simulink model "VCU_CS75_10_9_SteeringTorque"  (R2014a)
settings: Solver=FixedStepDiscrete  StartTime=0.0  StopTime=25  FixedStep=0.0005  RelTol=1e-3
undefined symbols (not defined in the file or in its folder): AutoDrivingReady, ecucoder_acal, I_SW01_L, LaterlAngleCommand, LDW, RemoteAcclPosition
libraries: simulink x880, ec5744lib x37
(part 22 of 30)

== system VCU_CS75_10_9_SteeringTorque/长安CS75底盘程序，20ms一次/Output/Subsystem/TransmitMessages4/ACC_3E5/ACC_takeoverRequesr ==
  ACC_takeoverRequesr : Inport
  ACC_takeoverRequesrRon : Rounding  Operator=round
  ACC_takeoverRequesr_1sat : Saturate  UpperLimit=8  LowerLimit=0
  ACC_takeoverRequesr_Convert : DataTypeConversion  OutDataTypeStr=uint8
  ACC_takeoverRequesr_Convert1 : DataTypeConversion  OutDataTypeStr=uint32
  ACC_takeoverRequesr_D : Product  Inputs=*/
  ACC_takeoverRequesr_F : Constant  OutDataTypeStr=single
  ACC_takeoverRequesr_L : simulink/Logic and Bit Operations/Bitwise Operator  logicop=AND  UseBitMask=on  BitMask=8  BitMaskRealWorld=Stored Integer
  ACC_takeoverRequesr_O : Constant  Value=0  OutDataTypeStr=single
  ACC_takeoverRequesr_S : ArithShift  BitShiftNumber=-3
  ACC_takeoverRequesr_sat : Saturate  UpperLimit=1  LowerLimit=0
  ACC_takeoverRequesr_st : Sum  Inputs=+-
  Constant{1..3,5..8} (7 alike) : Constant  Value=0  OutDataTypeStr=uint8
  output1 : Outport
  output2 : Outport  Port=2
  output3 : Outport  Port=3
  output4 : Outport  Port=4
  output5 : Outport  Port=5
  output6 : Outport  Port=6
  output7 : Outport  Port=7
  output8 : Outport  Port=8
  wires:
  Constant8/1 -> output8/1
  Constant7/1 -> output7/1
  Constant6/1 -> output6/1
  Constant5/1 -> output5/1
  Constant3/1 -> output3/1
  Constant2/1 -> output2/1
  Constant1/1 -> output1/1
  ACC_takeoverRequesr_Convert/1 -> output4/1
  ACC_takeoverRequesr_L/1 -> ACC_takeoverRequesr_Convert/1
  ACC_takeoverRequesr_Convert1/1 -> ACC_takeoverRequesr_L/1
  ACC_takeoverRequesr_1sat/1 -> ACC_takeoverRequesr_Convert1/1
  ACC_takeoverRequesr_S/1 -> ACC_takeoverRequesr_1sat/1
  ACC_takeoverRequesrRon/1 -> ACC_takeoverRequesr_S/1
  ACC_takeoverRequesr_D/1 -> ACC_takeoverRequesrRon/1
  ACC_takeoverRequesr_F/1 -> ACC_takeoverRequesr_D/2
  ACC_takeoverRequesr_st/1 -> ACC_takeoverRequesr_D/1
  ACC_takeoverRequesr_O/1 -> ACC_takeoverRequesr_st/2
  ACC_takeoverRequesr_sat/1 -> ACC_takeoverRequesr_st/1
  ACC_takeoverRequesr/1 -> ACC_takeoverRequesr_sat/1

== system VCU_CS75_10_9_SteeringTorque/长安CS75底盘程序，20ms一次/Output/Subsystem/TransmitMessages4/ACC_3E5/CRC ==
  CRC : Inport
  CRCRon : Rounding  Operator=round
  CRC_1sat : Saturate  UpperLimit=255  LowerLimit=0
  CRC_Convert : DataTypeConversion  OutDataTypeStr=uint8
  CRC_Convert1 : DataTypeConversion  OutDataTypeStr=uint32
  CRC_D : Product  Inputs=*/
  CRC_F : Constant  OutDataTypeStr=single
  CRC_L : simulink/Logic and Bit Operations/Bitwise Operator  logicop=AND  UseBitMask=on  BitMask=255  BitMaskRealWorld=Stored Integer
  CRC_O : Constant  Value=0  OutDataTypeStr=single
  CRC_S : ArithShift
  CRC_sat : Saturate  UpperLimit=0  LowerLimit=0
  CRC_st : Sum  Inputs=+-
  Constant{1..7} (7 alike) : Constant  Value=0  OutDataTypeStr=uint8
  output1 : Outport
  output2 : Outport  Port=2
  output3 : Outport  Port=3
  output4 : Outport  Port=4
  output5 : Outport  Port=5
  output6 : Outport  Port=6
  output7 : Outport  Port=7
  output8 : Outport  Port=8
  wires:
  Constant7/1 -> output7/1
  Constant6/1 -> output6/1
  Constant5/1 -> output5/1
  Constant4/1 -> output4/1
  Constant3/1 -> output3/1
  Constant2/1 -> output2/1
  Constant1/1 -> output1/1
  CRC_Convert/1 -> output8/1
  CRC_L/1 -> CRC_Convert/1
  CRC_Convert1/1 -> CRC_L/1
  CRC_1sat/1 -> CRC_Convert1/1
  CRC_S/1 -> CRC_1sat/1
  CRCRon/1 -> CRC_S/1
  CRC_D/1 -> CRCRon/1
  CRC_F/1 -> CRC_D/2
  CRC_st/1 -> CRC_D/1
  CRC_O/1 -> CRC_st/2
  CRC_sat/1 -> CRC_st/1
  CRC/1 -> CRC_sat/1

== system VCU_CS75_10_9_SteeringTorque/长安CS75底盘程序，20ms一次/Output/Subsystem/TransmitMessages4/ACC_3E5/RollingConter ==
  RollingConter : Inport
  Constant{1..6,8} (7 alike) : Constant  Value=0  OutDataTypeStr=uint8
  RollingConterRon : Rounding  Operator=round
  RollingConter_1sat : Saturate  UpperLimit=15  LowerLimit=0
  RollingConter_Convert : DataTypeConversion  OutDataTypeStr=uint8
  RollingConter_Convert1 : DataTypeConversion  OutDataTypeStr=uint32
  RollingConter_D : Product  Inputs=*/
  RollingConter_F : Constant  OutDataTypeStr=single
  RollingConter_L : simulink/Logic and Bit Operations/Bitwise Operator  logicop=AND  UseBitMask=on  BitMask=15  BitMaskRealWorld=Stored Integer
  RollingConter_O : Constant  Value=0  OutDataTypeStr=single
  RollingConter_S : ArithShift
  RollingConter_sat : Saturate  UpperLimit=0  LowerLimit=0
  RollingConter_st : Sum  Inputs=+-
  output1 : Outport
  output2 : Outport  Port=2
  output3 : Outport  Port=3
  output4 : Outport  Port=4
  output5 : Outport  Port=5
  output6 : Outport  Port=6
  output7 : Outport  Port=7
  output8 : Outport  Port=8
  wires:
  Constant8/1 -> output8/1
  Constant6/1 -> output6/1
  Constant5/1 -> output5/1
  Constant4/1 -> output4/1
  Constant3/1 -> output3/1
  Constant2/1 -> output2/1
  Constant1/1 -> output1/1
  RollingConter_Convert/1 -> output7/1
  RollingConter_L/1 -> RollingConter_Convert/1
  RollingConter_Convert1/1 -> RollingConter_L/1
  RollingConter_1sat/1 -> RollingConter_Convert1/1
  RollingConter_S/1 -> RollingConter_1sat/1
  RollingConterRon/1 -> RollingConter_S/1
  RollingConter_D/1 -> RollingConterRon/1
  RollingConter_F/1 -> RollingConter_D/2
  RollingConter_st/1 -> RollingConter_D/1
  RollingConter_O/1 -> RollingConter_st/2
  RollingConter_sat/1 -> RollingConter_st/1
  RollingConter/1 -> RollingConter_sat/1

== system VCU_CS75_10_9_SteeringTorque/长安CS75底盘程序，20ms一次/Output/Subsystem/TransmitMessages5/ACC_3F5/ACC_AEBTargetLatRange ==
  ACC_AEBTargetLatRange : Inport
  ACC_AEBTargetLatRangeBitCov : DataTypeConversion  OutDataTypeStr=uint8
  ACC_AEBTargetLatRangeCOV : DataTypeConversion  OutDataTypeStr=uint8
  ACC_AEBTargetLatRangeRon : Rounding  Operator=round
  ACC_AEBTargetLatRange_1sat : Saturate  UpperLimit=16368  LowerLimit=0
  ACC_AEBTargetLatRange_And : simulink/Logic and Bit Operations/Bitwise Operator  logicop=AND  UseBitMask=off  NumInputPorts=2  BitMask=bin2dec('11011001')  BitMaskRealWorld=Stored Integer
  ACC_AEBTargetLatRange_And_C : Constant  Value=255  OutDataTypeStr=uint32
  ACC_AEBTargetLatRange_Convert : DataTypeConversion  OutDataTypeStr=uint32
  ACC_AEBTargetLatRange_D : Product  Inputs=*/
  ACC_AEBTargetLatRange_D1 : Product  Inputs=*/
  ACC_AEBTargetLatRange_F : Constant  Value=0.1  OutDataTypeStr=single
  ACC_AEBTargetLatRange_L : simulink/Logic and Bit Operations/Bitwise Operator  logicop=AND  UseBitMask=on  BitMask=16368  BitMaskRealWorld=Stored Integer
  ACC_AEBTargetLatRange_O : Constant  Value=-50  OutDataTypeStr=single
  ACC_AEBTargetLatRange_S : ArithShift  BitShiftNumber=-4
  ACC_AEBTargetLatRange_sat : Saturate  UpperLimit=52.3  LowerLimit=-50
  ACC_AEBTargetLatRange_st : Sum  Inputs=+-
  ACC_AEBTargetLatRangeoutput3_C : Constant  Value=256
  Constant{1..2,5..8} (6 alike) : Constant  Value=0  OutDataTypeStr=uint8
  output1 : Outport
  output2 : Outport  Port=2
  output3 : Outport  Port=3
  output4 : Outport  Port=4
  output5 : Outport  Port=5
  output6 : Outport  Port=6
  output7 : Outport  Port=7
  output8 : Outport  Port=8
  wires:
  ACC_AEBTargetLatRange/1 -> ACC_AEBTargetLatRange_sat/1
  ACC_AEBTargetLatRange_sat/1 -> ACC_AEBTargetLatRange_st/1
  ACC_AEBTargetLatRange_O/1 -> ACC_AEBTargetLatRange_st/2
  ACC_AEBTargetLatRange_st/1 -> ACC_AEBTargetLatRange_D/1
  ACC_AEBTargetLatRange_F/1 -> ACC_AEBTargetLatRange_D/2
  ACC_AEBTargetLatRange_D/1 -> ACC_AEBTargetLatRangeRon/1
  ACC_AEBTargetLatRangeRon/1 -> ACC_AEBTargetLatRange_S/1
  ACC_AEBTargetLatRange_S/1 -> ACC_AEBTargetLatRange_1sat/1
  ACC_AEBTargetLatRange_1sat/1 -> ACC_AEBTargetLatRange_Convert/1
  ACC_AEBTargetLatRange_Convert/1 -> ACC_AEBTargetLatRange_L/1
  ACC_AEBTargetLatRange_L/1 -> ACC_AEBTargetLatRange_D1/1, ACC_AEBTargetLatRange_And/1
  ACC_AEBTargetLatRangeoutput3_C/1 -> ACC_AEBTargetLatRange_D1/2
  ACC_AEBTargetLatRange_D1/1 -> ACC_AEBTargetLatRangeCOV/1
  ACC_AEBTargetLatRangeCOV/1 -> output3/1
  ACC_AEBTargetLatRange_And_C/1 -> ACC_AEBTargetLatRange_And/2
  ACC_AEBTargetLatRange_And/1 -> ACC_AEBTargetLatRangeBitCov/1
  ACC_AEBTargetLatRangeBitCov/1 -> output4/1
  Constant1/1 -> output1/1
  Constant2/1 -> output2/1
  Constant5/1 -> output5/1
  Constant6/1 -> output6/1
  Constant7/1 -> output7/1
  Constant8/1 -> output8/1

== system VCU_CS75_10_9_SteeringTorque/长安CS75底盘程序，20ms一次/Output/Subsystem/TransmitMessages5/ACC_3F5/ACC_AEBTargetLngRange ==
  ACC_AEBTargetLngRange : Inport
  ACC_AEBTargetLngRangeBitCov : DataTypeConversion  OutDataTypeStr=uint8
  ACC_AEBTargetLngRangeCOV : DataTypeConversion  OutDataTypeStr=uint8
  ACC_AEBTargetLngRangeRon : Rounding  Operator=round
  ACC_AEBTargetLngRange_1sat : Saturate  UpperLimit=65408  LowerLimit=0
  ACC_AEBTargetLngRange_And : simulink/Logic and Bit Operations/Bitwise Operator  logicop=AND  UseBitMask=off  NumInputPorts=2  BitMask=bin2dec('11011001')  BitMaskRealWorld=Stored Integer
  ACC_AEBTargetLngRange_And_C : Constant  Value=255  OutDataTypeStr=uint32
  ACC_AEBTargetLngRange_Convert : DataTypeConversion  OutDataTypeStr=uint32
  ACC_AEBTargetLngRange_D : Product  Inputs=*/
  ACC_AEBTargetLngRange_D1 : Product  Inputs=*/
  ACC_AEBTargetLngRange_F : Constant  Value=0.5  OutDataTypeStr=single
  ACC_AEBTargetLngRange_L : simulink/Logic and Bit Operations/Bitwise Operator  logicop=AND  UseBitMask=on  BitMask=65408  BitMaskRealWorld=Stored Integer
  ACC_AEBTargetLngRange_O : Constant  Value=0  OutDataTypeStr=single
  ACC_AEBTargetLngRange_S : ArithShift  BitShiftNumber=-7
  ACC_AEBTargetLngRange_sat : Saturate  UpperLimit=0  LowerLimit=0
  ACC_AEBTargetLngRange_st : Sum  Inputs=+-
  ACC_AEBTargetLngRangeoutput1_C : Constant  Value=256
  Constant{3..8} (6 alike) : Constant  Value=0  OutDataTypeStr=uint8
  output1 : Outport
  output2 : Outport  Port=2
  output3 : Outport  Port=3
  output4 : Outport  Port=4
  output5 : Outport  Port=5
  output6 : Outport  Port=6
  output7 : Outport  Port=7
  output8 : Outport  Port=8
  wires:
  ACC_AEBTargetLngRange/1 -> ACC_AEBTargetLngRange_sat/1
  ACC_AEBTargetLngRange_sat/1 -> ACC_AEBTargetLngRange_st/1
  ACC_AEBTargetLngRange_O/1 -> ACC_AEBTargetLngRange_st/2
  ACC_AEBTargetLngRange_st/1 -> ACC_AEBTargetLngRange_D/1
  ACC_AEBTargetLngRange_F/1 -> ACC_AEBTargetLngRange_D/2
  ACC_AEBTargetLngRange_D/1 -> ACC_AEBTargetLngRangeRon/1
  ACC_AEBTargetLngRangeRon/1 -> ACC_AEBTargetLngRange_S/1
  ACC_AEBTargetLngRange_S/1 -> ACC_AEBTargetLngRange_1sat/1
  ACC_AEBTargetLngRange_1sat/1 -> ACC_AEBTargetLngRange_Convert/1
  ACC_AEBTargetLngRange_Convert/1 -> ACC_AEBTargetLngRange_L/1
  ACC_AEBTargetLngRange_L/1 -> ACC_AEBTargetLngRange_D1/1, ACC_AEBTargetLngRange_And/1
  ACC_AEBTargetLngRangeoutput1_C/1 -> ACC_AEBTargetLngRange_D1/2
  ACC_AEBTargetLngRange_D1/1 -> ACC_AEBTargetLngRangeCOV/1
  ACC_AEBTargetLngRangeCOV/1 -> output1/1
  ACC_AEBTargetLngRange_And_C/1 -> ACC_AEBTargetLngRange_And/2
  ACC_AEBTargetLngRange_And/1 -> ACC_AEBTargetLngRangeBitCov/1
  ACC_AEBTargetLngRangeBitCov/1 -> output2/1
  Constant3/1 -> output3/1
  Constant4/1 -> output4/1
  Constant5/1 -> output5/1
  Constant6/1 -> output6/1
  Constant7/1 -> output7/1
  Constant8/1 -> output8/1

== system VCU_CS75_10_9_SteeringTorque/长安CS75底盘程序，20ms一次/Output/Subsystem/TransmitMessages5/ACC_3F5/ACC_AEBTargetRelSpeed ==
  ACC_AEBTargetRelSpeed : Inport
  ACC_AEBTargetRelSpeedBitCov : DataTypeConversion  OutDataTypeStr=uint8
  ACC_AEBTargetRelSpeedCOV : DataTypeConversion  OutDataTypeStr=uint8
  ACC_AEBTargetRelSpeedRon : Rounding  Operator=round
  ACC_AEBTargetRelSpeed_1sat : Saturate  UpperLimit=32704  LowerLimit=0
  ACC_AEBTargetRelSpeed_And : simulink/Logic and Bit Operations/Bitwise Operator  logicop=AND  UseBitMask=off  NumInputPorts=2  BitMask=bin2dec('11011001')  BitMaskRealWorld=Stored Integer
  ACC_AEBTargetRelSpeed_And_C : Constant  Value=255  OutDataTypeStr=uint32
  ACC_AEBTargetRelSpeed_Convert : DataTypeConversion  OutDataTypeStr=uint32
  ACC_AEBTargetRelSpeed_D : Product  Inputs=*/
  ACC_AEBTargetRelSpeed_D1 : Product  Inputs=*/
  ACC_AEBTargetRelSpeed_F : Constant  OutDataTypeStr=single
  ACC_AEBTargetRelSpeed_L : simulink/Logic and Bit Operations/Bitwise Operator  logicop=AND  UseBitMask=on  BitMask=32704  BitMaskRealWorld=Stored Integer
  ACC_AEBTargetRelSpeed_O : Constant  Value=0  OutDataTypeStr=single
  ACC_AEBTargetRelSpeed_S : ArithShift  BitShiftNumber=-6
  ACC_AEBTargetRelSpeed_sat : Saturate  UpperLimit=0  LowerLimit=0
  ACC_AEBTargetRelSpeed_st : Sum  Inputs=+-
  ACC_AEBTargetRelSpeedoutput2_C : Constant  Value=256
  Constant{1,4..8} (6 alike) : Constant  Value=0  OutDataTypeStr=uint8
  output1 : Outport
  output2 : Outport  Port=2
  output3 : Outport  Port=3
  output4 : Outport  Port=4
  output5 : Outport  Port=5
  output6 : Outport  Port=6
  output7 : Outport  Port=7
  output8 : Outport  Port=8
  wires:
  ACC_AEBTargetRelSpeed/1 -> ACC_AEBTargetRelSpeed_sat/1
  ACC_AEBTargetRelSpeed_sat/1 -> ACC_AEBTargetRelSpeed_st/1
  ACC_AEBTargetRelSpeed_O/1 -> ACC_AEBTargetRelSpeed_st/2
  ACC_AEBTargetRelSpeed_st/1 -> ACC_AEBTargetRelSpeed_D/1
  ACC_AEBTargetRelSpeed_F/1 -> ACC_AEBTargetRelSpeed_D/2
  ACC_AEBTargetRelSpeed_D/1 -> ACC_AEBTargetRelSpeedRon/1
  ACC_AEBTargetRelSpeedRon/1 -> ACC_AEBTargetRelSpeed_S/1
  ACC_AEBTargetRelSpeed_S/1 -> ACC_AEBTargetRelSpeed_1sat/1
  ACC_AEBTargetRelSpeed_1sat/1 -> ACC_AEBTargetRelSpeed_Convert/1
  ACC_AEBTargetRelSpeed_Convert/1 -> ACC_AEBTargetRelSpeed_L/1
  ACC_AEBTargetRelSpeed_L/1 -> ACC_AEBTargetRelSpeed_D1/1, ACC_AEBTargetRelSpeed_And/1
  ACC_AEBTargetRelSpeedoutput2_C/1 -> ACC_AEBTargetRelSpeed_D1/2
  ACC_AEBTargetRelSpeed_D1/1 -> ACC_AEBTargetRelSpeedCOV/1
  ACC_AEBTargetRelSpeedCOV/1 -> output2/1
  ACC_AEBTargetRelSpeed_And_C/1 -> ACC_AEBTargetRelSpeed_And/2
  ACC_AEBTargetRelSpeed_And/1 -> ACC_AEBTargetRelSpeedBitCov/1
  ACC_AEBTargetRelSpeedBitCov/1 -> output3/1
  Constant1/1 -> output1/1
  Constant4/1 -> output4/1
  Constant5/1 -> output5/1
  Constant6/1 -> output6/1
  Constant7/1 -> output7/1
  Constant8/1 -> output8/1

== system VCU_CS75_10_9_SteeringTorque/长安CS75底盘程序，20ms一次/Output/Subsystem/TransmitMessages5/ACC_3F5/ACC_HostPotentialTargetDetection ==
  ACC_HostPotentialTargetDetection : Inport
  ACC_HostPotentialTargetDetectionRon : Rounding  Operator=round
  ACC_HostPotentialTargetDetection_1sat : Saturate  UpperLimit=12  LowerLimit=0
  ACC_HostPotentialTargetDetection_Convert : DataTypeConversion  OutDataTypeStr=uint8
  ACC_HostPotentialTargetDetection_Convert1 : DataTypeConversion  OutDataTypeStr=uint32
  ACC_HostPotentialTargetDetection_D : Product  Inputs=*/
  ACC_HostPotentialTargetDetection_F : Constant  OutDataTypeStr=single
  ACC_HostPotentialTargetDetection_L : simulink/Logic and Bit Operations/Bitwise Operator  logicop=AND  UseBitMask=on  BitMask=12  BitMaskRealWorld=Stored Integer
  ACC_HostPotentialTargetDetection_O : Constant  Value=0  OutDataTypeStr=single
  ACC_HostPotentialTargetDetection_S : ArithShift  BitShiftNumber=-2
  ACC_HostPotentialTargetDetection_sat : Saturate  UpperLimit=3  LowerLimit=0
  ACC_HostPotentialTargetDetection_st : Sum  Inputs=+-
  Constant{1..3,5..8} (7 alike) : Constant  Value=0  OutDataTypeStr=uint8
  output1 : Outport
  output2 : Outport  Port=2
  output3 : Outport  Port=3
  output4 : Outport  Port=4
  output5 : Outport  Port=5
  output6 : Outport  Port=6
  output7 : Outport  Port=7
  output8 : Outport  Port=8
  wires:
  ACC_HostPotentialTargetDetection/1 -> ACC_HostPotentialTargetDetection_sat/1
  ACC_HostPotentialTargetDetection_sat/1 -> ACC_HostPotentialTargetDetection_st/1
  ACC_HostPotentialTargetDetection_O/1 -> ACC_HostPotentialTargetDetection_st/2
  ACC_HostPotentialTargetDetection_st/1 -> ACC_HostPotentialTargetDetection_D/1
  ACC_HostPotentialTargetDetection_F/1 -> ACC_HostPotentialTargetDetection_D/2
  ACC_HostPotentialTargetDetection_D/1 -> ACC_HostPotentialTargetDetectionRon/1
  ACC_HostPotentialTargetDetectionRon/1 -> ACC_HostPotentialTargetDetection_S/1
  ACC_HostPotentialTargetDetection_S/1 -> ACC_HostPotentialTargetDetection_1sat/1
  ACC_HostPotentialTargetDetection_1sat/1 -> ACC_HostPotentialTargetDetection_Convert1/1
  ACC_HostPotentialTargetDetection_Convert1/1 -> ACC_HostPotentialTargetDetection_L/1
  ACC_HostPotentialTargetDetection_L/1 -> ACC_HostPotentialTargetDetection_Convert/1
  ACC_HostPotentialTargetDetection_Convert/1 -> output4/1
  Constant1/1 -> output1/1
  Constant2/1 -> output2/1
  Constant3/1 -> output3/1
  Constant5/1 -> output5/1
  Constant6/1 -> output6/1
  Constant7/1 -> output7/1
  Constant8/1 -> output8/1

== system VCU_CS75_10_9_SteeringTorque/长安CS75底盘程序，20ms一次/Output/Subsystem/TransmitMessages5/ACC_3F5/ACC_HostPotentialTargetLatRng ==
  ACC_HostPotentialTargetLatRng : Inport
  ACC_HostPotentialTargetLatRngBitCov : DataTypeConversion  OutDataTypeStr=uint8
  ACC_HostPotentialTargetLatRngCOV : DataTypeConversion  OutDataTypeStr=uint8
  ACC_HostPotentialTargetLatRngRon : Rounding  Operator=round
  ACC_HostPotentialTargetLatRng_1sat : Saturate  UpperLimit=1023  LowerLimit=0
  ACC_HostPotentialTargetLatRng_And : simulink/Logic and Bit Operations/Bitwise Operator  logicop=AND  UseBitMask=off  NumInputPorts=2  BitMask=bin2dec('11011001')  BitMaskRealWorld=Stored Integer
  ACC_HostPotentialTargetLatRng_And_C : Constant  Value=255  OutDataTypeStr=uint32
  ACC_HostPotentialTargetLatRng_Convert : DataTypeConversion  OutDataTypeStr=uint32
  ACC_HostPotentialTargetLatRng_D : Product  Inputs=*/
  ACC_HostPotentialTargetLatRng_D1 : Product  Inputs=*/
  ACC_HostPotentialTargetLatRng_F : Constant  Value=0.1  OutDataTypeStr=single
  ACC_HostPotentialTargetLatRng_L : simulink/Logic and Bit Operations/Bitwise Operator  logicop=AND  UseBitMask=on  BitMask=1023  BitMaskRealWorld=Stored Integer
  ACC_HostPotentialTargetLatRng_O : Constant  Value=-50  OutDataTypeStr=single
  ACC_HostPotentialTargetLatRng_S : ArithShift
  ACC_HostPotentialTargetLatRng_sat : Saturate  UpperLimit=52.3  LowerLimit=-50
  ACC_HostPotentialTargetLatRng_st : Sum  Inputs=+-
  ACC_HostPotentialTargetLatRngoutput4_C : Constant  Value=256
  Constant{1..3,6..8} (6 alike) : Constant  Value=0  OutDataTypeStr=uint8
  output1 : Outport
  output2 : Outport  Port=2
  output3 : Outport  Port=3
  output4 : Outport  Port=4
  output5 : Outport  Port=5
  output6 : Outport  Port=6
  output7 : Outport  Port=7
  output8 : Outport  Port=8
  wires:
  ACC_HostPotentialTargetLatRng/1 -> ACC_HostPotentialTargetLatRng_sat/1
  ACC_HostPotentialTargetLatRng_sat/1 -> ACC_HostPotentialTargetLatRng_st/1
  ACC_HostPotentialTargetLatRng_O/1 -> ACC_HostPotentialTargetLatRng_st/2
  ACC_HostPotentialTargetLatRng_st/1 -> ACC_HostPotentialTargetLatRng_D/1
  ACC_HostPotentialTargetLatRng_F/1 -> ACC_HostPotentialTargetLatRng_D/2
  ACC_HostPotentialTargetLatRng_D/1 -> ACC_HostPotentialTargetLatRngRon/1
  ACC_HostPotentialTargetLatRngRon/1 -> ACC_HostPotentialTargetLatRng_S/1
  ACC_HostPotentialTargetLatRng_S/1 -> ACC_HostPotentialTargetLatRng_1sat/1
  ACC_HostPotentialTargetLatRng_1sat/1 -> ACC_HostPotentialTargetLatRng_Convert/1
  ACC_HostPotentialTargetLatRng_Convert/1 -> ACC_HostPotentialTargetLatRng_L/1
  ACC_HostPotentialTargetLatRng_L/1 -> ACC_HostPotentialTargetLatRng_D1/1, ACC_HostPotentialTargetLatRng_And/1
  ACC_HostPotentialTargetLatRngoutput4_C/1 -> ACC_HostPotentialTargetLatRng_D1/2
  ACC_HostPotentialTargetLatRng_D1/1 -> ACC_HostPotentialTargetLatRngCOV/1
  ACC_HostPotentialTargetLatRngCOV/1 -> output4/1
  ACC_HostPotentialTargetLatRng_And_C/1 -> ACC_HostPotentialTargetLatRng_And/2
  ACC_HostPotentialTargetLatRng_And/1 -> ACC_HostPotentialTargetLatRngBitCov/1
  ACC_HostPotentialTargetLatRngBitCov/1 -> output5/1
  Constant1/1 -> output1/1
  Constant2/1 -> output2/1
  Constant3/1 -> output3/1
  Constant6/1 -> output6/1
  Constant7/1 -> output7/1
  Constant8/1 -> output8/1

== system VCU_CS75_10_9_SteeringTorque/长安CS75底盘程序，20ms一次/Output/Subsystem/TransmitMessages5/ACC_3F5/ACC_HostPotentialTargetLngRng ==
  ACC_HostPotentialTargetLngRng : Inport
  ACC_HostPotentialTargetLngRngBitCov : DataTypeConversion  OutDataTypeStr=uint8
  ACC_HostPotentialTargetLngRngCOV : DataTypeConversion  OutDataTypeStr=uint8
  ACC_HostPotentialTargetLngRngRon : Rounding  Operator=round
  ACC_HostPotentialTargetLngRng_1sat : Saturate  UpperLimit=65408  LowerLimit=0
  ACC_HostPotentialTargetLngRng_And : simulink/Logic and Bit Operations/Bitwise Operator  logicop=AND  UseBitMask=off  NumInputPorts=2  BitMask=bin2dec('11011001')  BitMaskRealWorld=Stored Integer
  ACC_HostPotentialTargetLngRng_And_C : Constant  Value=255  OutDataTypeStr=uint32
  ACC_HostPotentialTargetLngRng_Convert : DataTypeConversion  OutDataTypeStr=uint32
  ACC_HostPotentialTargetLngRng_D : Product  Inputs=*/
  ACC_HostPotentialTargetLngRng_D1 : Product  Inputs=*/
  ACC_HostPotentialTargetLngRng_F : Constant  Value=0.5  OutDataTypeStr=single
  ACC_HostPotentialTargetLngRng_L : simulink/Logic and Bit Operations/Bitwise Operator  logicop=AND  UseBitMask=on  BitMask=65408  BitMaskRealWorld=Stored Integer
  ACC_HostPotentialTargetLngRng_O : Constant  Value=0  OutDataTypeStr=single
  ACC_HostPotentialTargetLngRng_S : ArithShift  BitShiftNumber=-7
  ACC_HostPotentialTargetLngRng_sat : Saturate  UpperLimit=255.5  LowerLimit=0
  ACC_HostPotentialTargetLngRng_st : Sum  Inputs=+-
  ACC_HostPotentialTargetLngRngoutput6_C : Constant  Value=256
  Constant{1..5,8} (6 alike) : Constant  Value=0  OutDataTypeStr=uint8
  output1 : Outport
  output2 : Outport  Port=2
  output3 : Outport  Port=3
  output4 : Outport  Port=4
  output5 : Outport  Port=5
  output6 : Outport  Port=6
  output7 : Outport  Port=7
  output8 : Outport  Port=8
  wires:
  ACC_HostPotentialTargetLngRng/1 -> ACC_HostPotentialTargetLngRng_sat/1
  ACC_HostPotentialTargetLngRng_sat/1 -> ACC_HostPotentialTargetLngRng_st/1
  ACC_HostPotentialTargetLngRng_O/1 -> ACC_HostPotentialTargetLngRng_st/2
  ACC_HostPotentialTargetLngRng_st/1 -> ACC_HostPotentialTargetLngRng_D/1
  ACC_HostPotentialTargetLngRng_F/1 -> ACC_HostPotentialTargetLngRng_D/2
  ACC_HostPotentialTargetLngRng_D/1 -> ACC_HostPotentialTargetLngRngRon/1
  ACC_HostPotentialTargetLngRngRon/1 -> ACC_HostPotentialTargetLngRng_S/1
  ACC_HostPotentialTargetLngRng_S/1 -> ACC_HostPotentialTargetLngRng_1sat/1
  ACC_HostPotentialTargetLngRng_1sat/1 -> ACC_HostPotentialTargetLngRng_Convert/1
  ACC_HostPotentialTargetLngRng_Convert/1 -> ACC_HostPotentialTargetLngRng_L/1
  ACC_HostPotentialTargetLngRng_L/1 -> ACC_HostPotentialTargetLngRng_D1/1, ACC_HostPotentialTargetLngRng_And/1
  ACC_HostPotentialTargetLngRngoutput6_C/1 -> ACC_HostPotentialTargetLngRng_D1/2
  ACC_HostPotentialTargetLngRng_D1/1 -> ACC_HostPotentialTargetLngRngCOV/1
  ACC_HostPotentialTargetLngRngCOV/1 -> output6/1
  ACC_HostPotentialTargetLngRng_And_C/1 -> ACC_HostPotentialTargetLngRng_And/2
  ACC_HostPotentialTargetLngRng_And/1 -> ACC_HostPotentialTargetLngRngBitCov/1
  ACC_HostPotentialTargetLngRngBitCov/1 -> output7/1
  Constant1/1 -> output1/1
  Constant2/1 -> output2/1
  Constant3/1 -> output3/1
  Constant4/1 -> output4/1
  Constant5/1 -> output5/1
  Constant8/1 -> output8/1

== system VCU_CS75_10_9_SteeringTorque/长安CS75底盘程序，20ms一次/Output/Subsystem/TransmitMessages5/ACC_3F5/ACC_HostPotentialTargetType ==
  ACC_HostPotentialTargetType : Inport
  ACC_HostPotentialTargetTypeRon : Rounding  Operator=round
  ACC_HostPotentialTargetType_1sat : Saturate  UpperLimit=112  LowerLimit=0
  ACC_HostPotentialTargetType_Convert : DataTypeConversion  OutDataTypeStr=uint8
  ACC_HostPotentialTargetType_Convert1 : DataTypeConversion  OutDataTypeStr=uint32
  ACC_HostPotentialTargetType_D : Product  Inputs=*/
  ACC_HostPotentialTargetType_F : Constant  OutDataTypeStr=single
  ACC_HostPotentialTargetType_L : simulink/Logic and Bit Operations/Bitwise Operator  logicop=AND  UseBitMask=on  BitMask=112  BitMaskRealWorld=Stored Integer
  ACC_HostPotentialTargetType_O : Constant  Value=0  OutDataTypeStr=single
  ACC_HostPotentialTargetType_S : ArithShift  BitShiftNumber=-4
  ACC_HostPotentialTargetType_sat : Saturate  UpperLimit=7  LowerLimit=0
  ACC_HostPotentialTargetType_st : Sum  Inputs=+-
  Constant{1..6,8} (7 alike) : Constant  Value=0  OutDataTypeStr=uint8
  output1 : Outport
  output2 : Outport  Port=2
  output3 : Outport  Port=3
  output4 : Outport  Port=4
  output5 : Outport  Port=5
  output6 : Outport  Port=6
  output7 : Outport  Port=7
  output8 : Outport  Port=8
  wires:
  ACC_HostPotentialTargetType/1 -> ACC_HostPotentialTargetType_sat/1
  ACC_HostPotentialTargetType_sat/1 -> ACC_HostPotentialTargetType_st/1
  ACC_HostPotentialTargetType_O/1 -> ACC_HostPotentialTargetType_st/2
  ACC_HostPotentialTargetType_st/1 -> ACC_HostPotentialTargetType_D/1
  ACC_HostPotentialTargetType_F/1 -> ACC_HostPotentialTargetType_D/2
  ACC_HostPotentialTargetType_D/1 -> ACC_HostPotentialTargetTypeRon/1
  ACC_HostPotentialTargetTypeRon/1 -> ACC_HostPotentialTargetType_S/1
  ACC_HostPotentialTargetType_S/1 -> ACC_HostPotentialTargetType_1sat/1
  ACC_HostPotentialTargetType_1sat/1 -> ACC_HostPotentialTargetType_Convert1/1
  ACC_HostPotentialTargetType_Convert1/1 -> ACC_HostPotentialTargetType_L/1
  ACC_HostPotentialTargetType_L/1 -> ACC_HostPotentialTargetType_Convert/1
  ACC_HostPotentialTargetType_Convert/1 -> output7/1
  Constant1/1 -> output1/1
  Constant2/1 -> output2/1
  Constant3/1 -> output3/1
  Constant4/1 -> output4/1
  Constant5/1 -> output5/1
  Constant6/1 -> output6/1
  Constant8/1 -> output8/1

== system VCU_CS75_10_9_SteeringTorque/长安CS75底盘程序，20ms一次/Output/Subsystem/TransmitMessages5/ACC_3F5/CRC ==
  CRC : Inport
  CRCRon : Rounding  Operator=round
  CRC_1sat : Saturate  UpperLimit=255  LowerLimit=0
  CRC_Convert : DataTypeConversion  OutDataTypeStr=uint8
  CRC_Convert1 : DataTypeConversion  OutDataTypeStr=uint32
  CRC_D : Product  Inputs=*/
  CRC_F : Constant  OutDataTypeStr=single
  CRC_L : simulink/Logic and Bit Operations/Bitwise Operator  logicop=AND  UseBitMask=on  BitMask=255  BitMaskRealWorld=Stored Integer
  CRC_O : Constant  Value=0  OutDataTypeStr=single
  CRC_S : ArithShift
  CRC_sat : Saturate  UpperLimit=0  LowerLimit=0
  CRC_st : Sum  Inputs=+-
  Constant{1..7} (7 alike) : Constant  Value=0  OutDataTypeStr=uint8
  output1 : Outport
  output2 : Outport  Port=2
  output3 : Outport  Port=3
  output4 : Outport  Port=4
  output5 : Outport  Port=5
  output6 : Outport  Port=6
  output7 : Outport  Port=7
  output8 : Outport  Port=8
  wires:
  CRC/1 -> CRC_sat/1
  CRC_sat/1 -> CRC_st/1
  CRC_O/1 -> CRC_st/2
  CRC_st/1 -> CRC_D/1
  CRC_F/1 -> CRC_D/2
  CRC_D/1 -> CRCRon/1
  CRCRon/1 -> CRC_S/1
  CRC_S/1 -> CRC_1sat/1
  CRC_1sat/1 -> CRC_Convert1/1
  CRC_Convert1/1 -> CRC_L/1
  CRC_L/1 -> CRC_Convert/1
  CRC_Convert/1 -> output8/1
  Constant1/1 -> output1/1
  Constant2/1 -> output2/1
  Constant3/1 -> output3/1
  Constant4/1 -> output4/1
  Constant5/1 -> output5/1
  Constant6/1 -> output6/1
  Constant7/1 -> output7/1

== system VCU_CS75_10_9_SteeringTorque/长安CS75底盘程序，20ms一次/Output/Subsystem/TransmitMessages5/ACC_3F5/RollingConter ==
  RollingConter : Inport
  Constant{1..6,8} (7 alike) : Constant  Value=0  OutDataTypeStr=uint8
  RollingConterRon : Rounding  Operator=round
  RollingConter_1sat : Saturate  UpperLimit=15  LowerLimit=0
  RollingConter_Convert : DataTypeConversion  OutDataTypeStr=uint8
  RollingConter_Convert1 : DataTypeConversion  OutDataTypeStr=uint32
  RollingConter_D : Product  Inputs=*/
  RollingConter_F : Constant  OutDataTypeStr=single
  RollingConter_L : simulink/Logic and Bit Operations/Bitwise Operator  logicop=AND  UseBitMask=on  BitMask=15  BitMaskRealWorld=Stored Integer
  RollingConter_O : Constant  Value=0  OutDataTypeStr=single
  RollingConter_S : ArithShift
  RollingConter_sat : Saturate  UpperLimit=0  LowerLimit=0
  RollingConter_st : Sum  Inputs=+-
  output1 : Outport
  output2 : Outport  Port=2
  output3 : Outport  Port=3
  output4 : Outport  Port=4
  output5 : Outport  Port=5
  output6 : Outport  Port=6
  output7 : Outport  Port=7
  output8 : Outport  Port=8
  wires:
  RollingConter/1 -> RollingConter_sat/1
  RollingConter_sat/1 -> RollingConter_st/1
  RollingConter_O/1 -> RollingConter_st/2
  RollingConter_st/1 -> RollingConter_D/1
  RollingConter_F/1 -> RollingConter_D/2
  RollingConter_D/1 -> RollingConterRon/1
  RollingConterRon/1 -> RollingConter_S/1
  RollingConter_S/1 -> RollingConter_1sat/1
  RollingConter_1sat/1 -> RollingConter_Convert1/1
  RollingConter_Convert1/1 -> RollingConter_L/1
  RollingConter_L/1 -> RollingConter_Convert/1
  RollingConter_Convert/1 -> output7/1
  Constant1/1 -> output1/1
  Constant2/1 -> output2/1
  Constant3/1 -> output3/1
  Constant4/1 -> output4/1
  Constant5/1 -> output5/1
  Constant6/1 -> output6/1
  Constant8/1 -> output8/1

== system VCU_CS75_10_9_SteeringTorque/长安CS75底盘程序，20ms一次/Output/Subsystem/TransmitMessages7/APA_29A/APA_ActivationStatus ==
  APA_ActivationStatus : Inport
  APA_ActivationStatusRon : Rounding  Operator=round
  APA_ActivationStatus_1sat : Saturate  UpperLimit=224  LowerLimit=0
  APA_ActivationStatus_Convert : DataTypeConversion  OutDataTypeStr=uint8
  APA_ActivationStatus_Convert1 : DataTypeConversion  OutDataTypeStr=uint32
  APA_ActivationStatus_D : Product  Inputs=*/
  APA_ActivationStatus_F : Constant  OutDataTypeStr=single
  APA_ActivationStatus_L : simulink/Logic and Bit Operations/Bitwise Operator  logicop=AND  UseBitMask=on  BitMask=224  BitMaskRealWorld=Stored Integer
  APA_ActivationStatus_O : Constant  Value=0  OutDataTypeStr=single
  APA_ActivationStatus_S : ArithShift  BitShiftNumber=-5
  APA_ActivationStatus_sat : Saturate  UpperLimit=7  LowerLimit=0
  APA_ActivationStatus_st : Sum  Inputs=+-
  Constant{1..5,7..8} (7 alike) : Constant  Value=0  OutDataTypeStr=uint8
  output1 : Outport
  output2 : Outport  Port=2
  output3 : Outport  Port=3
  output4 : Outport  Port=4
  output5 : Outport  Port=5
  output6 : Outport  Port=6
  output7 : Outport  Port=7
  output8 : Outport  Port=8
  wires:
  APA_ActivationStatus/1 -> APA_ActivationStatus_sat/1
  APA_ActivationStatus_sat/1 -> APA_ActivationStatus_st/1
  APA_ActivationStatus_O/1 -> APA_ActivationStatus_st/2
  APA_ActivationStatus_st/1 -> APA_ActivationStatus_D/1
  APA_ActivationStatus_F/1 -> APA_ActivationStatus_D/2
  APA_ActivationStatus_D/1 -> APA_ActivationStatusRon/1
  APA_ActivationStatusRon/1 -> APA_ActivationStatus_S/1
  APA_ActivationStatus_S/1 -> APA_ActivationStatus_1sat/1
  APA_ActivationStatus_1sat/1 -> APA_ActivationStatus_Convert1/1
  APA_ActivationStatus_Convert1/1 -> APA_ActivationStatus_L/1
  APA_ActivationStatus_L/1 -> APA_ActivationStatus_Convert/1
  APA_ActivationStatus_Convert/1 -> output6/1
  Constant1/1 -> output1/1
  Constant2/1 -> output2/1
  Constant3/1 -> output3/1
  Constant4/1 -> output4/1
  Constant5/1 -> output5/1
  Constant7/1 -> output7/1
  Constant8/1 -> output8/1

== system VCU_CS75_10_9_SteeringTorque/长安CS75底盘程序，20ms一次/Output/Subsystem/TransmitMessages7/APA_29A/APA_Checksum ==
  APA_Checksum : Inport
  APA_ChecksumRon : Rounding  Operator=round
  APA_Checksum_1sat : Saturate  UpperLimit=240  LowerLimit=0
  APA_Checksum_Convert : DataTypeConversion  OutDataTypeStr=uint8
  APA_Checksum_Convert1 : DataTypeConversion  OutDataTypeStr=uint32
  APA_Checksum_D : Product  Inputs=*/
  APA_Checksum_F : Constant  OutDataTypeStr=single
  APA_Checksum_L : simulink/Logic and Bit Operations/Bitwise Operator  logicop=AND  UseBitMask=on  BitMask=240  BitMaskRealWorld=Stored Integer
  APA_Checksum_O : Constant  Value=0  OutDataTypeStr=single
  APA_Checksum_S : ArithShift  BitShiftNumber=-4
  APA_Checksum_sat : Saturate  UpperLimit=0  LowerLimit=0
  APA_Checksum_st : Sum  Inputs=+-
  Constant{1..7} (7 alike) : Constant  Value=0  OutDataTypeStr=uint8
  output1 : Outport
  output2 : Outport  Port=2
  output3 : Outport  Port=3
  output4 : Outport  Port=4
  output5 : Outport  Port=5
  output6 : Outport  Port=6
  output7 : Outport  Port=7
  output8 : Outport  Port=8
  wires:
  APA_Checksum/1 -> APA_Checksum_sat/1
  APA_Checksum_sat/1 -> APA_Checksum_st/1
  APA_Checksum_O/1 -> APA_Checksum_st/2
  APA_Checksum_st/1 -> APA_Checksum_D/1
  APA_Checksum_F/1 -> APA_Checksum_D/2
  APA_Checksum_D/1 -> APA_ChecksumRon/1
  APA_ChecksumRon/1 -> APA_Checksum_S/1
  APA_Checksum_S/1 -> APA_Checksum_1sat/1
  APA_Checksum_1sat/1 -> APA_Checksum_Convert1/1
  APA_Checksum_Convert1/1 -> APA_Checksum_L/1
  APA_Checksum_L/1 -> APA_Checksum_Convert/1
  APA_Checksum_Convert/1 -> output8/1
  Constant1/1 -> output1/1
  Constant2/1 -> output2/1
  Constant3/1 -> output3/1
  Constant4/1 -> output4/1
  Constant5/1 -> output5/1
  Constant6/1 -> output6/1
  Constant7/1 -> output7/1

== system VCU_CS75_10_9_SteeringTorque/长安CS75底盘程序，20ms一次/Output/Subsystem/TransmitMessages7/APA_29A/APA_EPBrequest ==
  APA_EPBrequest : Inport
  APA_EPBrequestRon : Rounding  Operator=round
  APA_EPBrequest_1sat : Saturate  UpperLimit=3  LowerLimit=0
  APA_EPBrequest_Convert : DataTypeConversion  OutDataTypeStr=uint8
  APA_EPBrequest_Convert1 : DataTypeConversion  OutDataTypeStr=uint32
  APA_EPBrequest_D : Product  Inputs=*/
  APA_EPBrequest_F : Constant  OutDataTypeStr=single
  APA_EPBrequest_L : simulink/Logic and Bit Operations/Bitwise Operator  logicop=AND  UseBitMask=on  BitMask=3  BitMaskRealWorld=Stored Integer
  APA_EPBrequest_O : Constant  Value=0  OutDataTypeStr=single
  APA_EPBrequest_S : ArithShift
  APA_EPBrequest_sat : Saturate  UpperLimit=0  LowerLimit=0
  APA_EPBrequest_st : Sum  Inputs=+-
  Constant{2..8} (7 alike) : Constant  Value=0  OutDataTypeStr=uint8
  output1 : Outport
  output2 : Outport  Port=2
  output3 : Outport  Port=3
  output4 : Outport  Port=4
  output5 : Outport  Port=5
  output6 : Outport  Port=6
  output7 : Outport  Port=7
  output8 : Outport  Port=8
  wires:
  APA_EPBrequest/1 -> APA_EPBrequest_sat/1
  APA_EPBrequest_sat/1 -> APA_EPBrequest_st/1
  APA_EPBrequest_O/1 -> APA_EPBrequest_st/2
  APA_EPBrequest_st/1 -> APA_EPBrequest_D/1
  APA_EPBrequest_F/1 -> APA_EPBrequest_D/2
  APA_EPBrequest_D/1 -> APA_EPBrequestRon/1
  APA_EPBrequestRon/1 -> APA_EPBrequest_S/1
  APA_EPBrequest_S/1 -> APA_EPBrequest_1sat/1
  APA_EPBrequest_1sat/1 -> APA_EPBrequest_Convert1/1
  APA_EPBrequest_Convert1/1 -> APA_EPBrequest_L/1
  APA_EPBrequest_L/1 -> APA_EPBrequest_Convert/1
  APA_EPBrequest_Convert/1 -> output1/1
  Constant2/1 -> output2/1
  Constant3/1 -> output3/1
  Constant4/1 -> output4/1
  Constant5/1 -> output5/1
  Constant6/1 -> output6/1
  Constant7/1 -> output7/1
  Constant8/1 -> output8/1

== system VCU_CS75_10_9_SteeringTorque/长安CS75底盘程序，20ms一次/Output/Subsystem/TransmitMessages7/APA_29A/APA_EPBrequestValid ==
  APA_EPBrequestValid : Inport
  APA_EPBrequestValidRon : Rounding  Operator=round
  APA_EPBrequestValid_1sat : Saturate  UpperLimit=4  LowerLimit=0
  APA_EPBrequestValid_Convert : DataTypeConversion  OutDataTypeStr=uint8
  APA_EPBrequestValid_Convert1 : DataTypeConversion  OutDataTypeStr=uint32
  APA_EPBrequestValid_D : Product  Inputs=*/
  APA_EPBrequestValid_F : Constant  OutDataTypeStr=single
  APA_EPBrequestValid_L : simulink/Logic and Bit Operations/Bitwise Operator  logicop=AND  UseBitMask=on  BitMask=4  BitMaskRealWorld=Stored Integer
  APA_EPBrequestValid_O : Constant  Value=0  OutDataTypeStr=single
  APA_EPBrequestValid_S : ArithShift  BitShiftNumber=-2
  APA_EPBrequestValid_sat : Saturate  UpperLimit=0  LowerLimit=0
  APA_EPBrequestValid_st : Sum  Inputs=+-
  Constant{2..8} (7 alike) : Constant  Value=0  OutDataTypeStr=uint8
  output1 : Outport
  output2 : Outport  Port=2
  output3 : Outport  Port=3
  output4 : Outport  Port=4
  output5 : Outport  Port=5
  output6 : Outport  Port=6
  output7 : Outport  Port=7
  output8 : Outport  Port=8
  wires:
  APA_EPBrequestValid/1 -> APA_EPBrequestValid_sat/1
  APA_EPBrequestValid_sat/1 -> APA_EPBrequestValid_st/1
  APA_EPBrequestValid_O/1 -> APA_EPBrequestValid_st/2
  APA_EPBrequestValid_st/1 -> APA_EPBrequestValid_D/1
  APA_EPBrequestValid_F/1 -> APA_EPBrequestValid_D/2
  APA_EPBrequestValid_D/1 -> APA_EPBrequestValidRon/1
  APA_EPBrequestValidRon/1 -> APA_EPBrequestValid_S/1
  APA_EPBrequestValid_S/1 -> APA_EPBrequestValid_1sat/1
  APA_EPBrequestValid_1sat/1 -> APA_EPBrequestValid_Convert1/1
  APA_EPBrequestValid_Convert1/1 -> APA_EPBrequestValid_L/1
  APA_EPBrequestValid_L/1 -> APA_EPBrequestValid_Convert/1
  APA_EPBrequestValid_Convert/1 -> output1/1
  Constant2/1 -> output2/1
  Constant3/1 -> output3/1
  Constant4/1 -> output4/1
  Constant5/1 -> output5/1
  Constant6/1 -> output6/1
  Constant7/1 -> output7/1
  Constant8/1 -> output8/1

== system VCU_CS75_10_9_SteeringTorque/长安CS75底盘程序，20ms一次/Output/Subsystem/TransmitMessages7/APA_29A/APA_GearReqValid ==
  APA_GearReqValid : Inport
  APA_GearReqValidRon : Rounding  Operator=round
  APA_GearReqValid_1sat : Saturate  UpperLimit=4  LowerLimit=0
  APA_GearReqValid_Convert : DataTypeConversion  OutDataTypeStr=uint8
  APA_GearReqValid_Convert1 : DataTypeConversion  OutDataTypeStr=uint32
  APA_GearReqValid_D : Product  Inputs=*/
  APA_GearReqValid_F : Constant  OutDataTypeStr=single
  APA_GearReqValid_L : simulink/Logic and Bit Operations/Bitwise Operator  logicop=AND  UseBitMask=on  BitMask=4  BitMaskRealWorld=Stored Integer
  APA_GearReqValid_O : Constant  Value=0  OutDataTypeStr=single
  APA_GearReqValid_S : ArithShift  BitShiftNumber=-2
  APA_GearReqValid_sat : Saturate  UpperLimit=1  LowerLimit=0
  APA_GearReqValid_st : Sum  Inputs=+-
  Constant{1..3,5..8} (7 alike) : Constant  Value=0  OutDataTypeStr=uint8
  output1 : Outport
  output2 : Outport  Port=2
  output3 : Outport  Port=3
  output4 : Outport  Port=4
  output5 : Outport  Port=5
  output6 : Outport  Port=6
  output7 : Outport  Port=7
  output8 : Outport  Port=8
  wires:
  APA_GearReqValid/1 -> APA_GearReqValid_sat/1
  APA_GearReqValid_sat/1 -> APA_GearReqValid_st/1
  APA_GearReqValid_O/1 -> APA_GearReqValid_st/2
  APA_GearReqValid_st/1 -> APA_GearReqValid_D/1
  APA_GearReqValid_F/1 -> APA_GearReqValid_D/2
  APA_GearReqValid_D/1 -> APA_GearReqValidRon/1
  APA_GearReqValidRon/1 -> APA_GearReqValid_S/1
  APA_GearReqValid_S/1 -> APA_GearReqValid_1sat/1
  APA_GearReqValid_1sat/1 -> APA_GearReqValid_Convert1/1
  APA_GearReqValid_Convert1/1 -> APA_GearReqValid_L/1
  APA_GearReqValid_L/1 -> APA_GearReqValid_Convert/1
  APA_GearReqValid_Convert/1 -> output4/1
  Constant1/1 -> output1/1
  Constant2/1 -> output2/1
  Constant3/1 -> output3/1
  Constant5/1 -> output5/1
  Constant6/1 -> output6/1
  Constant7/1 -> output7/1
  Constant8/1 -> output8/1

== system VCU_CS75_10_9_SteeringTorque/长安CS75底盘程序，20ms一次/Output/Subsystem/TransmitMessages7/APA_29A/APA_LSCAction ==
  APA_LSCAction : Inport
  APA_LSCActionRon : Rounding  Operator=round
  APA_LSCAction_1sat : Saturate  UpperLimit=8  LowerLimit=0
  APA_LSCAction_Convert : DataTypeConversion  OutDataTypeStr=uint8
  APA_LSCAction_Convert1 : DataTypeConversion  OutDataTypeStr=uint32
  APA_LSCAction_D : Product  Inputs=*/
  APA_LSCAction_F : Constant  OutDataTypeStr=single
  APA_LSCAction_L : simulink/Logic and Bit Operations/Bitwise Operator  logicop=AND  UseBitMask=on  BitMask=8  BitMaskRealWorld=Stored Integer
  APA_LSCAction_O : Constant  Value=0  OutDataTypeStr=single
  APA_LSCAction_S : ArithShift  BitShiftNumber=-3
  APA_LSCAction_sat : Saturate  UpperLimit=0  LowerLimit=0
  APA_LSCAction_st : Sum  Inputs=+-
  Constant{1..3,5..8} (7 alike) : Constant  Value=0  OutDataTypeStr=uint8
  output1 : Outport
  output2 : Outport  Port=2
  output3 : Outport  Port=3
  output4 : Outport  Port=4
  output5 : Outport  Port=5
  output6 : Outport  Port=6
  output7 : Outport  Port=7
  output8 : Outport  Port=8
  wires:
  APA_LSCAction/1 -> APA_LSCAction_sat/1
  APA_LSCAction_sat/1 -> APA_LSCAction_st/1
  APA_LSCAction_O/1 -> APA_LSCAction_st/2
  APA_LSCAction_st/1 -> APA_LSCAction_D/1
  APA_LSCAction_F/1 -> APA_LSCAction_D/2
  APA_LSCAction_D/1 -> APA_LSCActionRon/1
  APA_LSCActionRon/1 -> APA_LSCAction_S/1
  APA_LSCAction_S/1 -> APA_LSCAction_1sat/1
  APA_LSCAction_1sat/1 -> APA_LSCAction_Convert1/1
  APA_LSCAction_Convert1/1 -> APA_LSCAction_L/1
  APA_LSCAction_L/1 -> APA_LSCAction_Convert/1
  APA_LSCAction_Convert/1 -> output4/1
  Constant1/1 -> output1/1
  Constant2/1 -> output2/1
  Constant3/1 -> output3/1
  Constant5/1 -> output5/1
  Constant6/1 -> output6/1
  Constant7/1 -> output7/1
  Constant8/1 -> output8/1

== system VCU_CS75_10_9_SteeringTorque/长安CS75底盘程序，20ms一次/Output/Subsystem/TransmitMessages7/APA_29A/APA_RollingCounter ==
  APA_RollingCounter : Inport
  APA_RollingCounterRon : Rounding  Operator=round
  APA_RollingCounter_1sat : Saturate  UpperLimit=15  LowerLimit=0
  APA_RollingCounter_Convert : DataTypeConversion  OutDataTypeStr=uint8
  APA_RollingCounter_Convert1 : DataTypeConversion  OutDataTypeStr=uint32
  APA_RollingCounter_D : Product  Inputs=*/
  APA_RollingCounter_F : Constant  OutDataTypeStr=single
  APA_RollingCounter_L : simulink/Logic and Bit Operations/Bitwise Operator  logicop=AND  UseBitMask=on  BitMask=15  BitMaskRealWorld=Stored Integer
  APA_RollingCounter_O : Constant  Value=0  OutDataTypeStr=single
  APA_RollingCounter_S : ArithShift
  APA_RollingCounter_sat : Saturate  UpperLimit=0  LowerLimit=0
  APA_RollingCounter_st : Sum  Inputs=+-
  Constant{1..7} (7 alike) : Constant  Value=0  OutDataTypeStr=uint8
  output1 : Outport
  output2 : Outport  Port=2
  output3 : Outport  Port=3
  output4 : Outport  Port=4
  output5 : Outport  Port=5
  output6 : Outport  Port=6
  output7 : Outport  Port=7
  output8 : Outport  Port=8
  wires:
  APA_RollingCounter/1 -> APA_RollingCounter_sat/1
  APA_RollingCounter_sat/1 -> APA_RollingCounter_st/1
  APA_RollingCounter_O/1 -> APA_RollingCounter_st/2
  APA_RollingCounter_st/1 -> APA_RollingCounter_D/1
  APA_RollingCounter_F/1 -> APA_RollingCounter_D/2
  APA_RollingCounter_D/1 -> APA_RollingCounterRon/1
  APA_RollingCounterRon/1 -> APA_RollingCounter_S/1
  APA_RollingCounter_S/1 -> APA_RollingCounter_1sat/1
  APA_RollingCounter_1sat/1 -> APA_RollingCounter_Convert1/1
  APA_RollingCounter_Convert1/1 -> APA_RollingCounter_L/1
  APA_RollingCounter_L/1 -> APA_RollingCounter_Convert/1
  APA_RollingCounter_Convert/1 -> output8/1
  Constant1/1 -> output1/1
  Constant2/1 -> output2/1
  Constant3/1 -> output3/1
  Constant4/1 -> output4/1
  Constant5/1 -> output5/1
  Constant6/1 -> output6/1
  Constant7/1 -> output7/1

== system VCU_CS75_10_9_SteeringTorque/长安CS75底盘程序，20ms一次/Output/Subsystem/TransmitMessages7/APA_29A/APA_TargetAcceleration ==
  APA_TargetAcceleration : Inport
  APA_TargetAccelerationBitCov : DataTypeConversion  OutDataTypeStr=uint8
  APA_TargetAccelerationCOV : DataTypeConversion  OutDataTypeStr=uint8
  APA_TargetAccelerationRon : Rounding  Operator=round
  APA_TargetAcceleration_1sat : Saturate  UpperLimit=16320  LowerLimit=0
  APA_TargetAcceleration_And : simulink/Logic and Bit Operations/Bitwise Operator  logicop=AND  UseBitMask=off  NumInputPorts=2  BitMask=bin2dec('11011001')  BitMaskRealWorld=Stored Integer
  APA_TargetAcceleration_And_C : Constant  Value=255  OutDataTypeStr=uint32
  APA_TargetAcceleration_Convert : DataTypeConversion  OutDataTypeStr=uint32
  APA_TargetAcceleration_D : Product  Inputs=*/
  APA_TargetAcceleration_D1 : Product  Inputs=*/
  APA_TargetAcceleration_F : Constant  Value=0.05  OutDataTypeStr=single
  APA_TargetAcceleration_L : simulink/Logic and Bit Operations/Bitwise Operator  logicop=AND  UseBitMask=on  BitMask=16320  BitMaskRealWorld=Stored Integer
  APA_TargetAcceleration_O : Constant  Value=-5  OutDataTypeStr=single
  APA_TargetAcceleration_S : ArithShift  BitShiftNumber=-6
  APA_TargetAcceleration_sat : Saturate  UpperLimit=0  LowerLimit=0
  APA_TargetAcceleration_st : Sum  Inputs=+-
  APA_TargetAccelerationoutput2_C : Constant  Value=256
  Constant{1,4..8} (6 alike) : Constant  Value=0  OutDataTypeStr=uint8
  output1 : Outport
  output2 : Outport  Port=2
  output3 : Outport  Port=3
  output4 : Outport  Port=4
  output5 : Outport  Port=5
  output6 : Outport  Port=6
  output7 : Outport  Port=7
  output8 : Outport  Port=8
  wires:
  APA_TargetAcceleration/1 -> APA_TargetAcceleration_sat/1
  APA_TargetAcceleration_sat/1 -> APA_TargetAcceleration_st/1
  APA_TargetAcceleration_O/1 -> APA_TargetAcceleration_st/2
  APA_TargetAcceleration_st/1 -> APA_TargetAcceleration_D/1
  APA_TargetAcceleration_F/1 -> APA_TargetAcceleration_D/2
  APA_TargetAcceleration_D/1 -> APA_TargetAccelerationRon/1
  APA_TargetAccelerationRon/1 -> APA_TargetAcceleration_S/1
  APA_TargetAcceleration_S/1 -> APA_TargetAcceleration_1sat/1
  APA_TargetAcceleration_1sat/1 -> APA_TargetAcceleration_Convert/1
  APA_TargetAcceleration_Convert/1 -> APA_TargetAcceleration_L/1
  APA_TargetAcceleration_L/1 -> APA_TargetAcceleration_D1/1, APA_TargetAcceleration_And/1
  APA_TargetAccelerationoutput2_C/1 -> APA_TargetAcceleration_D1/2
  APA_TargetAcceleration_D1/1 -> APA_TargetAccelerationCOV/1
  APA_TargetAccelerationCOV/1 -> output2/1
  APA_TargetAcceleration_And_C/1 -> APA_TargetAcceleration_And/2
  APA_TargetAcceleration_And/1 -> APA_TargetAccelerationBitCov/1
  APA_TargetAccelerationBitCov/1 -> output3/1
  Constant1/1 -> output1/1
  Constant4/1 -> output4/1
  Constant5/1 -> output5/1
  Constant6/1 -> output6/1
  Constant7/1 -> output7/1
  Constant8/1 -> output8/1

== system VCU_CS75_10_9_SteeringTorque/长安CS75底盘程序，20ms一次/Output/Subsystem/TransmitMessages7/APA_29A/APA_TargetAccelerationValid ==
  APA_TargetAccelerationValid : Inport
  APA_TargetAccelerationValidRon : Rounding  Operator=round
  APA_TargetAccelerationValid_1sat : Saturate  UpperLimit=64  LowerLimit=0
  APA_TargetAccelerationValid_Convert : DataTypeConversion  OutDataTypeStr=uint8
  APA_TargetAccelerationValid_Convert1 : DataTypeConversion  OutDataTypeStr=uint32
  APA_TargetAccelerationValid_D : Product  Inputs=*/
  APA_TargetAccelerationValid_F : Constant  OutDataTypeStr=single
  APA_TargetAccelerationValid_L : simulink/Logic and Bit Operations/Bitwise Operator  logicop=AND  UseBitMask=on  BitMask=64  BitMaskRealWorld=Stored Integer
  APA_TargetAccelerationValid_O : Constant  Value=0  OutDataTypeStr=single
  APA_TargetAccelerationValid_S : ArithShift  BitShiftNumber=-6
  APA_TargetAccelerationValid_sat : Saturate  UpperLimit=0  LowerLimit=0
  APA_TargetAccelerationValid_st : Sum  Inputs=+-
  Constant{1,3..8} (7 alike) : Constant  Value=0  OutDataTypeStr=uint8
  output1 : Outport
  output2 : Outport  Port=2
  output3 : Outport  Port=3
  output4 : Outport  Port=4
  output5 : Outport  Port=5
  output6 : Outport  Port=6
  output7 : Outport  Port=7
  output8 : Outport  Port=8
  wires:
  APA_TargetAccelerationValid/1 -> APA_TargetAccelerationValid_sat/1
  APA_TargetAccelerationValid_sat/1 -> APA_TargetAccelerationValid_st/1
  APA_TargetAccelerationValid_O/1 -> APA_TargetAccelerationValid_st/2
  APA_TargetAccelerationValid_st/1 -> APA_TargetAccelerationValid_D/1
  APA_TargetAccelerationValid_F/1 -> APA_TargetAccelerationValid_D/2
  APA_TargetAccelerationValid_D/1 -> APA_TargetAccelerationValidRon/1
  APA_TargetAccelerationValidRon/1 -> APA_TargetAccelerationValid_S/1
  APA_TargetAccelerationValid_S/1 -> APA_TargetAccelerationValid_1sat/1
  APA_TargetAccelerationValid_1sat/1 -> APA_TargetAccelerationValid_Convert1/1
  APA_TargetAccelerationValid_Convert1/1 -> APA_TargetAccelerationValid_L/1
  APA_TargetAccelerationValid_L/1 -> APA_TargetAccelerationValid_Convert/1
  APA_TargetAccelerationValid_Convert/1 -> output2/1
  Constant1/1 -> output1/1
  Constant3/1 -> output3/1
  Constant4/1 -> output4/1
  Constant5/1 -> output5/1
  Constant6/1 -> output6/1
  Constant7/1 -> output7/1
  Constant8/1 -> output8/1

== system VCU_CS75_10_9_SteeringTorque/长安CS75底盘程序，20ms一次/Output/Subsystem/TransmitMessages7/APA_29A/APA_TranShiftReqValid ==
  APA_TranShiftReqValid : Inport
  APA_TranShiftReqValidRon : Rounding  Operator=round
  APA_TranShiftReqValid_1sat : Saturate  UpperLimit=8  LowerLimit=0
  APA_TranShiftReqValid_Convert : DataTypeConversion  OutDataTypeStr=uint8
  APA_TranShiftReqValid_Convert1 : DataTypeConversion  OutDataTypeStr=uint32
  APA_TranShiftReqValid_D : Product  Inputs=*/
  APA_TranShiftReqValid_F : Constant  OutDataTypeStr=single
  APA_TranShiftReqValid_L : simulink/Logic and Bit Operations/Bitwise Operator  logicop=AND  UseBitMask=on  BitMask=8  BitMaskRealWorld=Stored Integer
  APA_TranShiftReqValid_O : Constant  Value=0  OutDataTypeStr=single
  APA_TranShiftReqValid_S : ArithShift  BitShiftNumber=-3
  APA_TranShiftReqValid_sat : Saturate  UpperLimit=1  LowerLimit=0
  APA_TranShiftReqValid_st : Sum  Inputs=+-
  Constant{2..8} (7 alike) : Constant  Value=0  OutDataTypeStr=uint8
  output1 : Outport
  output2 : Outport  Port=2
  output3 : Outport  Port=3
  output4 : Outport  Port=4
  output5 : Outport  Port=5
  output6 : Outport  Port=6
  output7 : Outport  Port=7
  output8 : Outport  Port=8
  wires:
  APA_TranShiftReqValid/1 -> APA_TranShiftReqValid_sat/1
  APA_TranShiftReqValid_sat/1 -> APA_TranShiftReqValid_st/1
  APA_TranShiftReqValid_O/1 -> APA_TranShiftReqValid_st/2
  APA_TranShiftReqValid_st/1 -> APA_TranShiftReqValid_D/1
  APA_TranShiftReqValid_F/1 -> APA_TranShiftReqValid_D/2
  APA_TranShiftReqValid_D/1 -> APA_TranShiftReqValidRon/1
  APA_TranShiftReqValidRon/1 -> APA_TranShiftReqValid_S/1
  APA_TranShiftReqValid_S/1 -> APA_TranShiftReqValid_1sat/1
  APA_TranShiftReqValid_1sat/1 -> APA_TranShiftReqValid_Convert1/1
  APA_TranShiftReqValid_Convert1/1 -> APA_TranShiftReqValid_L/1
  APA_TranShiftReqValid_L/1 -> APA_TranShiftReqValid_Convert/1
  APA_TranShiftReqValid_Convert/1 -> output1/1
  Constant2/1 -> output2/1
  Constant3/1 -> output3/1
  Constant4/1 -> output4/1
  Constant5/1 -> output5/1
  Constant6/1 -> output6/1
  Constant7/1 -> output7/1
  Constant8/1 -> output8/1
